simulink model "consigna_5_1"  (R2024b)
settings: Solver=VariableStepAuto  StartTime=0.0  StopTime=1  MaxStep=1e-4  RelTol=1e-3
InitFcn:
  | parametros
undefined symbols (not defined in the file or in its folder): alpha_cu, b_eq, b_l, b_m, C_ts, J_eq, J_l, J_m, k_l, L_d, L_ls, L_q, lambda_m, P_p, r, R_s_40, R_ts_amb, Temp_s_ref
(part 3 of 3)

== system consigna_5_1/Sistema linealizado por retroalimentación no lineal5/Subsistema físico no lineal/Subsistema mecánico completo ==
  T_m : Inport
  T_l : Inport  Port=2
  Gain : Gain  Gain=b_m + b_l / (r^2)
  Gain1 : Gain  Gain=1/r
  Gain2 : Gain  Gain=1/(J_m + J_l / r^2)
  Sum : Sum  Inputs=-+-
  omega_m(0) = 0 : Integrator
  theta_m(0) = 0 : Integrator
  theta_m(t) : Outport
  omega_m(t) : Outport  Port=2
  wires:
  Gain2/1 -> omega_m(0) = 0/1  "domega_m(t)/dt"
  Gain1/1 -> Sum/1
  theta_m(0) = 0/1 -> theta_m(t)/1  "theta_m(t)"
  omega_m(0) = 0/1 -> omega_m(t)/1, Gain/1, theta_m(0) = 0/1  "omega_m(t)"
  Sum/1 -> Gain2/1
  Gain/1 -> Sum/3
  T_l/1 -> Gain1/1
  T_m/1 -> Sum/2

== system consigna_5_1/Sistema linealizado por retroalimentación no lineal5/Subsistema físico no lineal/Subsistema térmico ==
  i_qs^r : Inport
  i_ds^r : Inport  Port=2
  i_0s^r : Inport  Port=3
  Tº_amb : Inport  Port=4
  Constant : Constant  Value=Temp_s_ref
  Constant1 : Constant
  Gain : Gain  Gain=1/C_ts
  Gain1 : Gain  Gain=3/2
  Gain2 : Gain  Gain=1/R_ts_amb
  Gain3 : Gain  Gain=alpha_cu
  Gain4 : Gain  Gain=R_s_40
  Gain5 : Gain  Gain=2
  Integrator : Integrator  InitialCondition=40
  Product : Product
  Square : Math  Operator=square
  Square1 : Math  Operator=square
  Square2 : Math  Operator=square
  Sum : Sum  Inputs=+++
  Sum1 : Sum  Inputs=-|+
  Sum2 : Sum  Inputs=|+-
  Sum3 : Sum  Inputs=|+-
  Sum4 : Sum  Inputs=|++
  r_s : Outport
  T_s : Outport  Port=2
  wires:
  i_qs^r/1 -> Square/1
  i_ds^r/1 -> Square1/1
  i_0s^r/1 -> Square2/1
  Gain/1 -> Integrator/1
  Square/1 -> Sum/1
  Square1/1 -> Sum/2
  Sum/1 -> Product/1
  Product/1 -> Gain1/1
  Tº_amb/1 -> Sum1/1
  Integrator/1 -> T_s/1, Sum3/1, Sum1/2
  Sum1/1 -> Gain2/1
  Gain1/1 -> Sum2/1
  Gain2/1 -> Sum2/2
  Sum2/1 -> Gain/1
  Constant/1 -> Sum3/2
  Sum3/1 -> Gain3/1
  Gain3/1 -> Sum4/1
  Constant1/1 -> Sum4/2
  Sum4/1 -> Gain4/1
  Gain4/1 -> Product/2, r_s/1
  Square2/1 -> Gain5/1
  Gain5/1 -> Sum/3

== system consigna_5_1/Sistema linealizado por retroalimentación no lineal6/Subsistema físico no lineal/Subsistema electromagnético ==
  v_qs^r : Inport
  v_ds^r : Inport  Port=2
  v_0s : Inport  Port=3
  r_s : Inport  Port=4
  omega_m : Inport  Port=5
  Gain : Gain  Gain=P_p
  Gain1 : Gain  Gain=L_d
  Gain2 : Gain  Gain=lambda_m
  Gain3 : Gain  Gain=1/L_q
  Gain4 : Gain  Gain=L_q
  Gain5 : Gain  Gain=1/L_d
  Gain6 : Gain  Gain=1/L_ls
  Gain7 : Gain  Gain=L_d-L_q
  Gain8 : Gain  Gain=lambda_m
  Gain9 : Gain  Gain=(3/2)*P_p
  Integrator : Integrator
  Integrator1 : Integrator
  Integrator2 : Integrator
  Product{,1..5} (6 alike) : Product
  Sum{,1..3,5} (5 alike) : Sum  Inputs=-+|
  Sum4 : Sum  Inputs=++|
  Sum6 : Sum  Inputs=++|
  i_qs^r : Outport
  i_ds^r : Outport  Port=2
  i_0s : Outport  Port=3
  T_m : Outport  Port=4
  wires:
  v_qs^r/1 -> Sum/2
  Product/1 -> Sum/1
  Sum/1 -> Sum1/2
  Integrator/1 -> Gain8/1, Product5/1, i_qs^r/1, Product/2, Gain4/1  "i_qs^r"
  omega_m/1 -> Gain/1
  Gain/1 -> Gain2/1, Product1/1, Product3/1
  Integrator1/1 -> Product2/2, Product5/2, i_ds^r/1, Gain1/1  "i_ds^r"
  Gain1/1 -> Product1/2
  Sum1/1 -> Sum2/2
  Sum2/1 -> Gain3/1
  Gain2/1 -> Sum2/1
  Product1/1 -> Sum1/1
  Gain3/1 -> Integrator/1
  Product2/1 -> Sum3/1
  v_ds^r/1 -> Sum3/2
  Sum3/1 -> Sum4/2
  Product3/1 -> Sum4/1
  Gain4/1 -> Product3/2
  Gain5/1 -> Integrator1/1
  Sum4/1 -> Gain5/1
  Integrator2/1 -> Product4/2, i_0s/1  "i_0s"
  r_s/1 -> Product4/1, Product/1, Product2/1
  Product4/1 -> Sum5/1
  v_0s/1 -> Sum5/2
  Sum5/1 -> Gain6/1
  Gain6/1 -> Integrator2/1
  Product5/1 -> Gain7/1
  Gain7/1 -> Sum6/2
  Gain8/1 -> Sum6/1
  Sum6/1 -> Gain9/1
  Gain9/1 -> T_m/1

== system consigna_5_1/Sistema linealizado por retroalimentación no lineal6/Subsistema físico no lineal/Subsistema mecánico completo ==
  T_m : Inport
  T_l : Inport  Port=2
  Gain : Gain  Gain=b_m + b_l / (r^2)
  Gain2 : Gain  Gain=1/(J_m + J_l / r^2)
  Gain3 : Gain  Gain=1/r
  Sum : Sum  Inputs=-+-
  omega_m(0) = 0 : Integrator
  theta_m(0) = 0 : Integrator
  theta_m(t) : Outport
  omega_m(t) : Outport  Port=2
  wires:
  Gain2/1 -> omega_m(0) = 0/1  "domega_m(t)/dt"
  T_l/1 -> Gain3/1
  theta_m(0) = 0/1 -> theta_m(t)/1  "theta_m(t)"
  omega_m(0) = 0/1 -> omega_m(t)/1, Gain/1, theta_m(0) = 0/1  "omega_m(t)"
  Sum/1 -> Gain2/1
  Gain/1 -> Sum/3
  T_m/1 -> Sum/2
  Gain3/1 -> Sum/1

== system consigna_5_1/Sistema linealizado por retroalimentación no lineal6/Subsistema físico no lineal/Subsistema térmico ==
  i_qs^r : Inport
  i_ds^r : Inport  Port=2
  i_0s^r : Inport  Port=3
  Tº_amb : Inport  Port=4
  Constant : Constant  Value=Temp_s_ref
  Constant1 : Constant
  Gain : Gain  Gain=1/C_ts
  Gain1 : Gain  Gain=3/2
  Gain2 : Gain  Gain=1/R_ts_amb
  Gain3 : Gain  Gain=alpha_cu
  Gain4 : Gain  Gain=R_s_40
  Gain5 : Gain  Gain=2
  Integrator : Integrator  InitialCondition=40
  Product : Product
  Square : Math  Operator=square
  Square1 : Math  Operator=square
  Square2 : Math  Operator=square
  Sum : Sum  Inputs=+++
  Sum1 : Sum  Inputs=-|+
  Sum2 : Sum  Inputs=|+-
  Sum3 : Sum  Inputs=|+-
  Sum4 : Sum  Inputs=|++
  r_s : Outport
  T_s : Outport  Port=2
  wires:
  i_qs^r/1 -> Square/1
  i_ds^r/1 -> Square1/1
  i_0s^r/1 -> Square2/1
  Gain/1 -> Integrator/1
  Square/1 -> Sum/1
  Square1/1 -> Sum/2
  Sum/1 -> Product/1
  Product/1 -> Gain1/1
  Tº_amb/1 -> Sum1/1
  Integrator/1 -> T_s/1, Sum3/1, Sum1/2
  Sum1/1 -> Gain2/1
  Gain1/1 -> Sum2/1
  Gain2/1 -> Sum2/2
  Sum2/1 -> Gain/1
  Constant/1 -> Sum3/2
  Sum3/1 -> Gain3/1
  Gain3/1 -> Sum4/1
  Constant1/1 -> Sum4/2
  Sum4/1 -> Gain4/1
  Gain4/1 -> Product/2, r_s/1
  Square2/1 -> Gain5/1
  Gain5/1 -> Sum/3

== matlab function consigna_5_1/Sistema linealizado por retroalimentación no lineal2/TD_PARK ==
  data: fas input; fqs output; fbs input; fcs input; theta_r input; fds output; f0s output
function [fqs, fds, f0s] = TD_PARK(fas, fbs, fcs, theta_r)

    fabcs = [fas; fbs; fcs];

    Ks = 2/3*[cos(theta_r) cos(theta_r - 2*pi/3) cos(theta_r + 2*pi/3)
          sin(theta_r) sin(theta_r - 2*pi/3) sin(theta_r + 2*pi/3) 
          1/2          1/2                   1/2];

    fqd0s = Ks * fabcs;

    fqs = fqd0s(1);
    fds = fqd0s(2);
    f0s = fqd0s(3);

end

== matlab function consigna_5_1/Sistema linealizado por retroalimentación no lineal2/TI_PARK ==
  data: fqs input; fas output; fds input; f0s input; theta_r input; fbs output; fcs output
function [fas, fbs, fcs] = TI_PARK(fqs, fds, f0s , theta_r)

    fqd0s = [fqs; fds; f0s];

    Ks = [cos(theta_r)         sin(theta_r)             1
          cos(theta_r - 2*pi/3) sin(theta_r - 2*pi/3)    1
          cos(theta_r + 2*pi/3) sin(theta_r + 2*pi/3)    1];

    fabcs = Ks * fqd0s;

    fas = fabcs(1);
    fbs = fabcs(2);
    fcs = fabcs(3);

end

== matlab function consigna_5_1/Sistema completo/Subsistema físico no lineal/TI_PARK ==
  data: fqs input; fas output; fds input; f0s input; theta_r input; fbs output; fcs output
function [fas, fbs, fcs] = TI_PARK(fqs, fds, f0s , theta_r)

    fqd0s = [fqs; fds; f0s];

    Ks = [cos(theta_r)         sin(theta_r)             1
          cos(theta_r - 2*pi/3) sin(theta_r - 2*pi/3)    1
          cos(theta_r + 2*pi/3) sin(theta_r + 2*pi/3)    1];

    fabcs = Ks * fqd0s;

    fas = fabcs(1);
    fbs = fabcs(2);
    fcs = fabcs(3);

end

== matlab function consigna_5_1/Sistema linealizado por retroalimentación no lineal1/Subsistema físico no lineal/TD_PARK ==
  data: fas input; fqs output; fbs input; fcs input; theta_r input; fds output; f0s output
function [fqs, fds, f0s] = TD_PARK(fas, fbs, fcs, theta_r)

    fabcs = [fas; fbs; fcs];

    Ks = 2/3*[cos(theta_r) cos(theta_r - 2*pi/3) cos(theta_r + 2*pi/3)
          sin(theta_r) sin(theta_r - 2*pi/3) sin(theta_r + 2*pi/3) 
          1/2          1/2                   1/2];

    fqd0s = Ks * fabcs;

    fqs = fqd0s(1);
    fds = fqd0s(2);
    f0s = fqd0s(3);

end

== matlab function consigna_5_1/Sistema linealizado por retroalimentación no lineal1/Subsistema físico no lineal/TI_PARK ==
  data: fqs input; fas output; fds input; f0s input; theta_r input; fbs output; fcs output
function [fas, fbs, fcs] = TI_PARK(fqs, fds, f0s , theta_r)

    fqd0s = [fqs; fds; f0s];

    Ks = [cos(theta_r)         sin(theta_r)             1
          cos(theta_r - 2*pi/3) sin(theta_r - 2*pi/3)    1
          cos(theta_r + 2*pi/3) sin(theta_r + 2*pi/3)    1];

    fabcs = Ks * fqd0s;

    fas = fabcs(1);
    fbs = fabcs(2);
    fcs = fabcs(3);

end

== matlab function consigna_5_1/Sistema linealizado por retroalimentación no lineal1/TD_PARK ==
  data: fas input; fqs output; fbs input; fcs input; theta_r input; fds output; f0s output
function [fqs, fds, f0s] = TD_PARK(fas, fbs, fcs, theta_r)

    fabcs = [fas; fbs; fcs];

    Ks = 2/3*[cos(theta_r) cos(theta_r - 2*pi/3) cos(theta_r + 2*pi/3)
          sin(theta_r) sin(theta_r - 2*pi/3) sin(theta_r + 2*pi/3) 
          1/2          1/2                   1/2];

    fqd0s = Ks * fabcs;

    fqs = fqd0s(1);
    fds = fqd0s(2);
    f0s = fqd0s(3);

end

== matlab function consigna_5_1/Sistema linealizado por retroalimentación no lineal1/TI_PARK ==
  data: fqs input; fas output; fds input; f0s input; theta_r input; fbs output; fcs output
function [fas, fbs, fcs] = TI_PARK(fqs, fds, f0s , theta_r)

    fqd0s = [fqs; fds; f0s];

    Ks = [cos(theta_r)         sin(theta_r)             1
          cos(theta_r - 2*pi/3) sin(theta_r - 2*pi/3)    1
          cos(theta_r + 2*pi/3) sin(theta_r + 2*pi/3)    1];

    fabcs = Ks * fqd0s;

    fas = fabcs(1);
    fbs = fabcs(2);
    fcs = fabcs(3);

end

== matlab function consigna_5_1/Sistema lineal equivalente3/TI_PARK ==
  data: fqs input; fas output; fds input; f0s input; theta_r input; fbs output; fcs output
function [fas, fbs, fcs] = TI_PARK(fqs, fds, f0s , theta_r)

    fqd0s = [fqs; fds; f0s];

    Ks = [cos(theta_r)         sin(theta_r)             1
          cos(theta_r - 2*pi/3) sin(theta_r - 2*pi/3)    1
          cos(theta_r + 2*pi/3) sin(theta_r + 2*pi/3)    1];

    fabcs = Ks * fqd0s;

    fas = fabcs(1);
    fbs = fabcs(2);
    fcs = fabcs(3);

end

== matlab function consigna_5_1/Sistema lineal equivalente3/TI_PARK1 ==
  data: fqs input; fas output; fds input; f0s input; theta_r input; fbs output; fcs output
function [fas, fbs, fcs] = TI_PARK(fqs, fds, f0s , theta_r)

    fqd0s = [fqs; fds; f0s];

    Ks = [cos(theta_r)         sin(theta_r)             1
          cos(theta_r - 2*pi/3) sin(theta_r - 2*pi/3)    1
          cos(theta_r + 2*pi/3) sin(theta_r + 2*pi/3)    1];

    fabcs = Ks * fqd0s;

    fas = fabcs(1);
    fbs = fabcs(2);
    fcs = fabcs(3);

end

== matlab function consigna_5_1/Sistema linealizado por retroalimentación no lineal3/Subsistema físico no lineal/TD_PARK ==
  data: fas input; fqs output; fbs input; fcs input; theta_r input; fds output; f0s output
function [fqs, fds, f0s] = TD_PARK(fas, fbs, fcs, theta_r)

    fabcs = [fas; fbs; fcs];

    Ks = 2/3*[cos(theta_r) cos(theta_r - 2*pi/3) cos(theta_r + 2*pi/3)
          sin(theta_r) sin(theta_r - 2*pi/3) sin(theta_r + 2*pi/3) 
          1/2          1/2                   1/2];

    fqd0s = Ks * fabcs;

    fqs = fqd0s(1);
    fds = fqd0s(2);
    f0s = fqd0s(3);

end

== matlab function consigna_5_1/Sistema linealizado por retroalimentación no lineal3/Subsistema físico no lineal/TI_PARK ==
  data: fqs input; fas output; fds input; f0s input; theta_r input; fbs output; fcs output
function [fas, fbs, fcs] = TI_PARK(fqs, fds, f0s , theta_r)

    fqd0s = [fqs; fds; f0s];

    Ks = [cos(theta_r)         sin(theta_r)             1
          cos(theta_r - 2*pi/3) sin(theta_r - 2*pi/3)    1
          cos(theta_r + 2*pi/3) sin(theta_r + 2*pi/3)    1];

    fabcs = Ks * fqd0s;

    fas = fabcs(1);
    fbs = fabcs(2);
    fcs = fabcs(3);

end

== matlab function consigna_5_1/Sistema linealizado por retroalimentación no lineal3/TD_PARK ==
  data: fas input; fqs output; fbs input; fcs input; theta_r input; fds output; f0s output
function [fqs, fds, f0s] = TD_PARK(fas, fbs, fcs, theta_r)

    fabcs = [fas; fbs; fcs];

    Ks = 2/3*[cos(theta_r) cos(theta_r - 2*pi/3) cos(theta_r + 2*pi/3)
          sin(theta_r) sin(theta_r - 2*pi/3) sin(theta_r + 2*pi/3) 
          1/2          1/2                   1/2];

    fqd0s = Ks * fabcs;

    fqs = fqd0s(1);
    fds = fqd0s(2);
    f0s = fqd0s(3);

end

== matlab function consigna_5_1/Sistema linealizado por retroalimentación no lineal3/TI_PARK ==
  data: fqs input; fas output; fds input; f0s input; theta_r input; fbs output; fcs output
function [fas, fbs, fcs] = TI_PARK(fqs, fds, f0s , theta_r)

    fqd0s = [fqs; fds; f0s];

    Ks = [cos(theta_r)         sin(theta_r)             1
          cos(theta_r - 2*pi/3) sin(theta_r - 2*pi/3)    1
          cos(theta_r + 2*pi/3) sin(theta_r + 2*pi/3)    1];

    fabcs = Ks * fqd0s;

    fas = fabcs(1);
    fbs = fabcs(2);
    fcs = fabcs(3);

end

== matlab function consigna_5_1/Sistema completo/Subsistema físico no lineal/TD_PARK ==
  data: fas input; fqs output; fbs input; fcs input; theta_r input; fds output; f0s output
function [fqs, fds, f0s] = TD_PARK(fas, fbs, fcs, theta_r)

    fabcs = [fas; fbs; fcs];

    Ks = 2/3*[cos(theta_r) cos(theta_r - 2*pi/3) cos(theta_r + 2*pi/3)
          sin(theta_r) sin(theta_r - 2*pi/3) sin(theta_r + 2*pi/3) 
          1/2          1/2                   1/2];

    fqd0s = Ks * fabcs;

    fqs = fqd0s(1);
    fds = fqd0s(2);
    f0s = fqd0s(3);

end

== matlab function consigna_5_1/Sistema linealizado por retroalimentación no lineal4/Subsistema físico no lineal/TD_PARK ==
  data: fas input; fqs output; fbs input; fcs input; theta_r input; fds output; f0s output
function [fqs, fds, f0s] = TD_PARK(fas, fbs, fcs, theta_r)

    fabcs = [fas; fbs; fcs];

    Ks = 2/3*[cos(theta_r) cos(theta_r - 2*pi/3) cos(theta_r + 2*pi/3)
          sin(theta_r) sin(theta_r - 2*pi/3) sin(theta_r + 2*pi/3) 
          1/2          1/2                   1/2];

    fqd0s = Ks * fabcs;

    fqs = fqd0s(1);
    fds = fqd0s(2);
    f0s = fqd0s(3);

end

== matlab function consigna_5_1/Sistema linealizado por retroalimentación no lineal4/Subsistema físico no lineal/TI_PARK ==
  data: fqs input; fas output; fds input; f0s input; theta_r input; fbs output; fcs output
function [fas, fbs, fcs] = TI_PARK(fqs, fds, f0s , theta_r)

    fqd0s = [fqs; fds; f0s];

    Ks = [cos(theta_r)         sin(theta_r)             1
          cos(theta_r - 2*pi/3) sin(theta_r - 2*pi/3)    1
          cos(theta_r + 2*pi/3) sin(theta_r + 2*pi/3)    1];

    fabcs = Ks * fqd0s;

    fas = fabcs(1);
    fbs = fabcs(2);
    fcs = fabcs(3);

end

== matlab function consigna_5_1/Sistema linealizado por retroalimentación no lineal4/TD_PARK ==
  data: fas input; fqs output; fbs input; fcs input; theta_r input; fds output; f0s output
function [fqs, fds, f0s] = TD_PARK(fas, fbs, fcs, theta_r)

    fabcs = [fas; fbs; fcs];

    Ks = 2/3*[cos(theta_r) cos(theta_r - 2*pi/3) cos(theta_r + 2*pi/3)
          sin(theta_r) sin(theta_r - 2*pi/3) sin(theta_r + 2*pi/3) 
          1/2          1/2                   1/2];

    fqd0s = Ks * fabcs;

    fqs = fqd0s(1);
    fds = fqd0s(2);
    f0s = fqd0s(3);

end

== matlab function consigna_5_1/Sistema linealizado por retroalimentación no lineal4/TI_PARK ==
  data: fqs input; fas output; fds input; f0s input; theta_r input; fbs output; fcs output
function [fas, fbs, fcs] = TI_PARK(fqs, fds, f0s , theta_r)

    fqd0s = [fqs; fds; f0s];

    Ks = [cos(theta_r)         sin(theta_r)             1
          cos(theta_r - 2*pi/3) sin(theta_r - 2*pi/3)    1
          cos(theta_r + 2*pi/3) sin(theta_r + 2*pi/3)    1];

    fabcs = Ks * fqd0s;

    fas = fabcs(1);
    fbs = fabcs(2);
    fcs = fabcs(3);

end

== matlab function consigna_5_1/Sistema linealizado por retroalimentación no lineal5/Subsistema físico no lineal/TD_PARK ==
  data: fas input; fqs output; fbs input; fcs input; theta_r input; fds output; f0s output
function [fqs, fds, f0s] = TD_PARK(fas, fbs, fcs, theta_r)

    fabcs = [fas; fbs; fcs];

    Ks = 2/3*[cos(theta_r) cos(theta_r - 2*pi/3) cos(theta_r + 2*pi/3)
          sin(theta_r) sin(theta_r - 2*pi/3) sin(theta_r + 2*pi/3) 
          1/2          1/2                   1/2];

    fqd0s = Ks * fabcs;

    fqs = fqd0s(1);
    fds = fqd0s(2);
    f0s = fqd0s(3);

end

== matlab function consigna_5_1/Sistema linealizado por retroalimentación no lineal5/Subsistema físico no lineal/TI_PARK ==
  data: fqs input; fas output; fds input; f0s input; theta_r input; fbs output; fcs output
function [fas, fbs, fcs] = TI_PARK(fqs, fds, f0s , theta_r)

    fqd0s = [fqs; fds; f0s];

    Ks = [cos(theta_r)         sin(theta_r)             1
          cos(theta_r - 2*pi/3) sin(theta_r - 2*pi/3)    1
          cos(theta_r + 2*pi/3) sin(theta_r + 2*pi/3)    1];

    fabcs = Ks * fqd0s;

    fas = fabcs(1);
    fbs = fabcs(2);
    fcs = fabcs(3);

end

== matlab function consigna_5_1/Sistema linealizado por retroalimentación no lineal5/TD_PARK ==
  data: fas input; fqs output; fbs input; fcs input; theta_r input; fds output; f0s output
function [fqs, fds, f0s] = TD_PARK(fas, fbs, fcs, theta_r)

    fabcs = [fas; fbs; fcs];

    Ks = 2/3*[cos(theta_r) cos(theta_r - 2*pi/3) cos(theta_r + 2*pi/3)
          sin(theta_r) sin(theta_r - 2*pi/3) sin(theta_r + 2*pi/3) 
          1/2          1/2                   1/2];

    fqd0s = Ks * fabcs;

    fqs = fqd0s(1);
    fds = fqd0s(2);
    f0s = fqd0s(3);

end

== matlab function consigna_5_1/Sistema linealizado por retroalimentación no lineal5/TI_PARK ==
  data: fqs input; fas output; fds input; f0s input; theta_r input; fbs output; fcs output
function [fas, fbs, fcs] = TI_PARK(fqs, fds, f0s , theta_r)

    fqd0s = [fqs; fds; f0s];

    Ks = [cos(theta_r)         sin(theta_r)             1
          cos(theta_r - 2*pi/3) sin(theta_r - 2*pi/3)    1
          cos(theta_r + 2*pi/3) sin(theta_r + 2*pi/3)    1];

    fabcs = Ks * fqd0s;

    fas = fabcs(1);
    fbs = fabcs(2);
    fcs = fabcs(3);

end

== matlab function consigna_5_1/Sistema linealizado por retroalimentación no lineal6/Subsistema físico no lineal/TD_PARK ==
  data: fas input; fqs output; fbs input; fcs input; theta_r input; fds output; f0s output
function [fqs, fds, f0s] = TD_PARK(fas, fbs, fcs, theta_r)

    fabcs = [fas; fbs; fcs];

    Ks = 2/3*[cos(theta_r) cos(theta_r - 2*pi/3) cos(theta_r + 2*pi/3)
          sin(theta_r) sin(theta_r - 2*pi/3) sin(theta_r + 2*pi/3) 
          1/2          1/2                   1/2];

    fqd0s = Ks * fabcs;

    fqs = fqd0s(1);
    fds = fqd0s(2);
    f0s = fqd0s(3);

end

== matlab function consigna_5_1/Sistema linealizado por retroalimentación no lineal6/Subsistema físico no lineal/TI_PARK ==
  data: fqs input; fas output; fds input; f0s input; theta_r input; fbs output; fcs output
function [fas, fbs, fcs] = TI_PARK(fqs, fds, f0s , theta_r)

    fqd0s = [fqs; fds; f0s];

    Ks = [cos(theta_r)         sin(theta_r)             1
          cos(theta_r - 2*pi/3) sin(theta_r - 2*pi/3)    1
          cos(theta_r + 2*pi/3) sin(theta_r + 2*pi/3)    1];

    fabcs = Ks * fqd0s;

    fas = fabcs(1);
    fbs = fabcs(2);
    fcs = fabcs(3);

end

== matlab function consigna_5_1/Sistema lineal equivalente1/TI_PARK ==
  data: fqs input; fas output; fds input; f0s input; theta_r input; fbs output; fcs output
function [fas, fbs, fcs] = TI_PARK(fqs, fds, f0s , theta_r)

    fqd0s = [fqs; fds; f0s];

    Ks = [cos(theta_r)         sin(theta_r)             1
          cos(theta_r - 2*pi/3) sin(theta_r - 2*pi/3)    1
          cos(theta_r + 2*pi/3) sin(theta_r + 2*pi/3)    1];

    fabcs = Ks * fqd0s;

    fas = fabcs(1);
    fbs = fabcs(2);
    fcs = fabcs(3);

end

== matlab function consigna_5_1/Sistema linealizado por retroalimentación no lineal6/TD_PARK ==
  data: fas input; fqs output; fbs input; fcs input; theta_r input; fds output; f0s output
function [fqs, fds, f0s] = TD_PARK(fas, fbs, fcs, theta_r)

    fabcs = [fas; fbs; fcs];

    Ks = 2/3*[cos(theta_r) cos(theta_r - 2*pi/3) cos(theta_r + 2*pi/3)
          sin(theta_r) sin(theta_r - 2*pi/3) sin(theta_r + 2*pi/3) 
          1/2          1/2                   1/2];

    fqd0s = Ks * fabcs;

    fqs = fqd0s(1);
    fds = fqd0s(2);
    f0s = fqd0s(3);

end

== matlab function consigna_5_1/Sistema linealizado por retroalimentación no lineal6/TI_PARK ==
  data: fqs input; fas output; fds input; f0s input; theta_r input; fbs output; fcs output
function [fas, fbs, fcs] = TI_PARK(fqs, fds, f0s , theta_r)

    fqd0s = [fqs; fds; f0s];

    Ks = [cos(theta_r)         sin(theta_r)             1
          cos(theta_r - 2*pi/3) sin(theta_r - 2*pi/3)    1
          cos(theta_r + 2*pi/3) sin(theta_r + 2*pi/3)    1];

    fabcs = Ks * fqd0s;

    fas = fabcs(1);
    fbs = fabcs(2);
    fcs = fabcs(3);

end

== matlab function consigna_5_1/Sistema lineal equivalente1/TI_PARK1 ==
  data: fqs input; fas output; fds input; f0s input; theta_r input; fbs output; fcs output
function [fas, fbs, fcs] = TI_PARK(fqs, fds, f0s , theta_r)

    fqd0s = [fqs; fds; f0s];

    Ks = [cos(theta_r)         sin(theta_r)             1
          cos(theta_r - 2*pi/3) sin(theta_r - 2*pi/3)    1
          cos(theta_r + 2*pi/3) sin(theta_r + 2*pi/3)    1];

    fabcs = Ks * fqd0s;

    fas = fabcs(1);
    fbs = fabcs(2);
    fcs = fabcs(3);

end

== matlab function consigna_5_1/Sistema lineal equivalente2/TI_PARK ==
  data: fqs input; fas output; fds input; f0s input; theta_r input; fbs output; fcs output
function [fas, fbs, fcs] = TI_PARK(fqs, fds, f0s , theta_r)

    fqd0s = [fqs; fds; f0s];

    Ks = [cos(theta_r)         sin(theta_r)             1
          cos(theta_r - 2*pi/3) sin(theta_r - 2*pi/3)    1
          cos(theta_r + 2*pi/3) sin(theta_r + 2*pi/3)    1];

    fabcs = Ks * fqd0s;

    fas = fabcs(1);
    fbs = fabcs(2);
    fcs = fabcs(3);

end

== matlab function consigna_5_1/Sistema lineal equivalente2/TI_PARK1 ==
  data: fqs input; fas output; fds input; f0s input; theta_r input; fbs output; fcs output
function [fas, fbs, fcs] = TI_PARK(fqs, fds, f0s , theta_r)

    fqd0s = [fqs; fds; f0s];

    Ks = [cos(theta_r)         sin(theta_r)             1
          cos(theta_r - 2*pi/3) sin(theta_r - 2*pi/3)    1
          cos(theta_r + 2*pi/3) sin(theta_r + 2*pi/3)    1];

    fabcs = Ks * fqd0s;

    fas = fabcs(1);
    fbs = fabcs(2);
    fcs = fabcs(3);

end

== matlab function consigna_5_1/Sistema linealizado por retroalimentación no lineal2/Subsistema físico no lineal/TD_PARK ==
  data: fas input; fqs output; fbs input; fcs input; theta_r input; fds output; f0s output
function [fqs, fds, f0s] = TD_PARK(fas, fbs, fcs, theta_r)

    fabcs = [fas; fbs; fcs];

    Ks = 2/3*[cos(theta_r) cos(theta_r - 2*pi/3) cos(theta_r + 2*pi/3)
          sin(theta_r) sin(theta_r - 2*pi/3) sin(theta_r + 2*pi/3) 
          1/2          1/2                   1/2];

    fqd0s = Ks * fabcs;

    fqs = fqd0s(1);
    fds = fqd0s(2);
    f0s = fqd0s(3);

end

== matlab function consigna_5_1/Sistema linealizado por retroalimentación no lineal2/Subsistema físico no lineal/TI_PARK ==
  data: fqs input; fas output; fds input; f0s input; theta_r input; fbs output; fcs output
function [fas, fbs, fcs] = TI_PARK(fqs, fds, f0s , theta_r)

    fqd0s = [fqs; fds; f0s];

    Ks = [cos(theta_r)         sin(theta_r)             1
          cos(theta_r - 2*pi/3) sin(theta_r - 2*pi/3)    1
          cos(theta_r + 2*pi/3) sin(theta_r + 2*pi/3)    1];

    fabcs = Ks * fqd0s;

    fas = fabcs(1);
    fbs = fabcs(2);
    fcs = fabcs(3);

end
